simulink model "exp03_sist_integro"  (Simulink 7.7)
settings: Solver=ode23t  StartTime=0.0  StopTime=0.1  RelTol=1e-5
libraries: powerlib x13, powerlib_extras x6
settings Model: Creator=alunos  LastModifiedBy=alunos

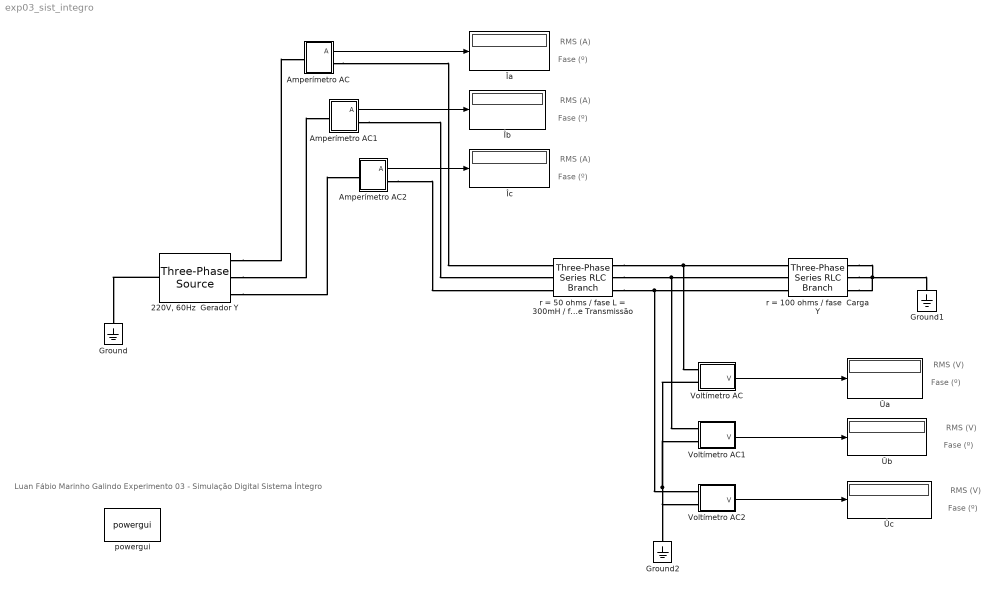
== system exp03_sist_integro ==
  note: RMS (A)
  note: Fase (º)
  note: RMS (A)
  note: Fase (º)
  note: RMS (A)
  note: Fase (º)
  note: RMS (V)
  note: Fase (º)
  note: RMS (V)
  note: Fase (º)
  note: RMS (V)
  note: Fase (º)
  note: Luan Fábio Marinho Galindo
      | Experimento 03 - Simulação Digital
      | Sistema Íntegro
  "220V, 60Hz  Gerador Y" : powerlib/Electrical Sources/Three-Phase Source  SystemSampleTime=-1  Voltage=220  PhaseAngle=90  Frequency=60  InternalConnection=Yn  SpecifyImpedance=off  Resistance=0.001  Inductance=0  ShortCircuitLevel=100e6  BaseVoltage=25e3  XRratio=7  BusType=swing  Pref=0  Qref=0  Qmin=-inf  Qmax=inf
  Amperímetro AC : Subsystem
  Amperímetro AC1 : Subsystem
  Amperímetro AC2 : Subsystem
  Ground : powerlib/Elements/Ground  PhysicalDomain=powersysdomain  SubClassName=unknown  LeftPortType=p1  RightPortType=p1  LConnTagsString=a
  Ground1 : powerlib/Elements/Ground  PhysicalDomain=powersysdomain  SubClassName=unknown  LeftPortType=p1  RightPortType=p1  LConnTagsString=a
  Ground2 : powerlib/Elements/Ground  PhysicalDomain=powersysdomain  SubClassName=unknown  LeftPortType=p1  RightPortType=p1  LConnTagsString=a
  Voltímetro AC : Subsystem
  Voltímetro AC1 : Subsystem
  Voltímetro AC2 : Subsystem
  powergui : powerlib/powergui  Priority=1  SystemSampleTime=-1  SimulationMode=Continuous  SampleTime=50e-6  frequency=60  SPID=off  DisableSnubberDevices=off  DisableRonSwitches=off  DisableVfSwitches=off  SwTol=0  Interpol=off  DisplayEquations=off  FunctionMessages=off  frequencyindice=60  Pbase=100e6  ErrMax=1e-4  Iterations=50  UnitsV=kV  UnitsW=MW  echomessages=off  HookPort=off  EnableUseOfTLC=off  x0status=blocks  RestoreLinks=warning  ResistiveCurrentMeasurement=off  Ylog=off  Xlog=on  ShowGrid=off  save=off  variable=ZData  ZoomFFT=off  StartTime=0.0  cycles=1  DisplayStyle=1  FreqAxis=off  MaxFrequency=1000  frequencyindicesteady=1  display=off  methode=off
  r = 100 ohms / fase  Carga Y : powerlib/Elements/Three-Phase Series RLC Branch  PhysicalDomain=powersysdomain  SubClassName=unknown  LeftPortType=p1  RightPortType=p1  LConnTagsString=A|B|C  RConnTagsString=A|B|C  BranchType=R  Resistance=100  Inductance=1e-3  Capacitance=1e-6  Measurements=None
  r = 50 ohms / fase L = 300mH / fase  Linha de Transmissão : powerlib/Elements/Three-Phase Series RLC Branch  PhysicalDomain=powersysdomain  SubClassName=unknown  LeftPortType=p1  RightPortType=p1  LConnTagsString=A|B|C  RConnTagsString=A|B|C  BranchType=RL  Resistance=50  Inductance=300e-3  Capacitance=1e-6  Measurements=None
  Îa : Display
      settings: Format=bank
  Îb : Display
      settings: Format=bank
  Îc : Display
      settings: Format=bank
  Ûa : Display
      settings: Format=bank
  Ûb : Display
      settings: Format=bank
  Ûc : Display
      settings: Format=bank
  wires:
  Amperímetro AC/1(A) -> Îa/1
  Amperímetro AC1/1(A) -> Îb/1
  Amperímetro AC2/1(A) -> Îc/1
  Voltímetro AC/1(V) -> Ûa/1
  Voltímetro AC1/1(V) -> Ûb/1
  Voltímetro AC2/1(V) -> Ûc/1
  connections:
  "220V, 60Hz  Gerador Y"/RConn1 -- Amperímetro AC/LConn1
  "220V, 60Hz  Gerador Y"/RConn2 -- Amperímetro AC1/LConn1
  "220V, 60Hz  Gerador Y"/RConn3 -- Amperímetro AC2/LConn1
  Amperímetro AC/RConn1 -- r = 50 ohms / fase L = 300mH / fase  Linha de Transmissão/LConn1
  Amperímetro AC1/RConn1 -- r = 50 ohms / fase L = 300mH / fase  Linha de Transmissão/LConn2
  Amperímetro AC2/RConn1 -- r = 50 ohms / fase L = 300mH / fase  Linha de Transmissão/LConn3
  r = 100 ohms / fase  Carga Y/RConn2 -- Ground1/LConn1 -- r = 100 ohms / fase  Carga Y/RConn3 -- r = 100 ohms / fase  Carga Y/RConn1
  r = 50 ohms / fase L = 300mH / fase  Linha de Transmissão/RConn1 -- r = 100 ohms / fase  Carga Y/LConn1 -- Voltímetro AC/LConn1
  r = 50 ohms / fase L = 300mH / fase  Linha de Transmissão/RConn2 -- r = 100 ohms / fase  Carga Y/LConn2 -- Voltímetro AC1/LConn1
  r = 50 ohms / fase L = 300mH / fase  Linha de Transmissão/RConn3 -- r = 100 ohms / fase  Carga Y/LConn3 -- Voltímetro AC2/LConn1
  Voltímetro AC/LConn2 -- Voltímetro AC1/LConn2 -- Ground2/LConn1 -- Voltímetro AC2/LConn2
  "220V, 60Hz  Gerador Y"/LConn1 -- Ground/LConn1

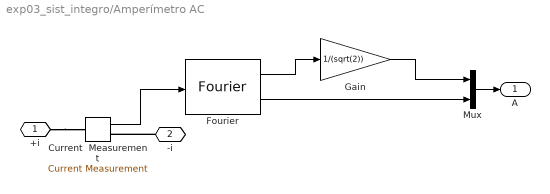
== system exp03_sist_integro/Amperímetro AC ==
  Current  Measurement : powerlib/Measurements/Current Measurement  SystemSampleTime=-1  PhasorSimulation=off  OutputType=Complex  PSBequivalent=0
  Fourier : powerlib_extras/Measurements/Fourier  SystemSampleTime=-1  f1=60  n=1
  Gain : Gain  Gain=1/(sqrt(2))
  Mux : Mux  Inputs=2
  +i : PMIOPort  Port=1  Side=Left
  -i : PMIOPort  Port=2  Side=Right
  A : Outport
  wires:
  Fourier/1 -> Gain/1
  Fourier/2 -> Mux/2
  Gain/1 -> Mux/1
  Current  Measurement/1 -> Fourier/1
  Mux/1 -> A/1
  connections:
  +i/RConn1 -- Current  Measurement/LConn1
  -i/RConn1 -- Current  Measurement/RConn1

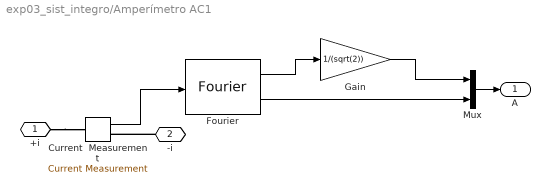
== system exp03_sist_integro/Amperímetro AC1 ==
  Current  Measurement : powerlib/Measurements/Current Measurement  SystemSampleTime=-1  PhasorSimulation=off  OutputType=Complex  PSBequivalent=0
  Fourier : powerlib_extras/Measurements/Fourier  SystemSampleTime=-1  f1=60  n=1
  Gain : Gain  Gain=1/(sqrt(2))
  Mux : Mux  Inputs=2
  +i : PMIOPort  Port=1  Side=Left
  -i : PMIOPort  Port=2  Side=Right
  A : Outport
  wires:
  Fourier/1 -> Gain/1
  Fourier/2 -> Mux/2
  Gain/1 -> Mux/1
  Current  Measurement/1 -> Fourier/1
  Mux/1 -> A/1
  connections:
  +i/RConn1 -- Current  Measurement/LConn1
  -i/RConn1 -- Current  Measurement/RConn1

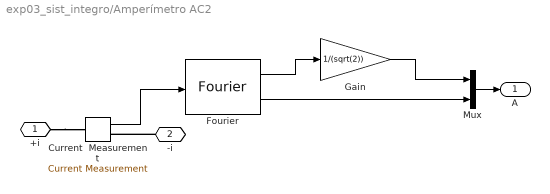
== system exp03_sist_integro/Amperímetro AC2 ==
  Current  Measurement : powerlib/Measurements/Current Measurement  SystemSampleTime=-1  PhasorSimulation=off  OutputType=Complex  PSBequivalent=0
  Fourier : powerlib_extras/Measurements/Fourier  SystemSampleTime=-1  f1=60  n=1
  Gain : Gain  Gain=1/(sqrt(2))
  Mux : Mux  Inputs=2
  +i : PMIOPort  Port=1  Side=Left
  -i : PMIOPort  Port=2  Side=Right
  A : Outport
  wires:
  Fourier/1 -> Gain/1
  Fourier/2 -> Mux/2
  Gain/1 -> Mux/1
  Current  Measurement/1 -> Fourier/1
  Mux/1 -> A/1
  connections:
  +i/RConn1 -- Current  Measurement/LConn1
  -i/RConn1 -- Current  Measurement/RConn1

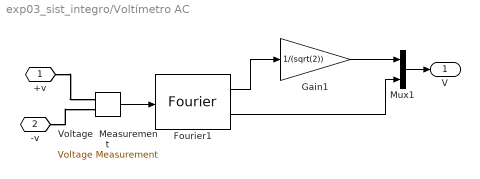
== system exp03_sist_integro/Voltímetro AC ==
  Fourier1 : powerlib_extras/Measurements/Fourier  SystemSampleTime=-1  f1=60  n=1
  Gain1 : Gain  Gain=1/(sqrt(2))
  Mux1 : Mux  Inputs=2
  Voltage  Measurement : powerlib/Measurements/Voltage Measurement  SystemSampleTime=-1  PhasorSimulation=off  OutputType=Complex  PSBequivalent=0
  +v : PMIOPort  Port=1  Side=Left
  -v : PMIOPort  Port=2  Side=Left
  V : Outport
  wires:
  Voltage  Measurement/1 -> Fourier1/1
  Fourier1/1 -> Gain1/1
  Gain1/1 -> Mux1/1
  Fourier1/2 -> Mux1/2
  Mux1/1 -> V/1
  connections:
  +v/RConn1 -- Voltage  Measurement/LConn1
  -v/RConn1 -- Voltage  Measurement/LConn2

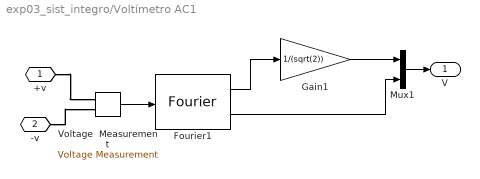
== system exp03_sist_integro/Voltímetro AC1 ==
  Fourier1 : powerlib_extras/Measurements/Fourier  SystemSampleTime=-1  f1=60  n=1
  Gain1 : Gain  Gain=1/(sqrt(2))
  Mux1 : Mux  Inputs=2
  Voltage  Measurement : powerlib/Measurements/Voltage Measurement  SystemSampleTime=-1  PhasorSimulation=off  OutputType=Complex  PSBequivalent=0
  +v : PMIOPort  Port=1  Side=Left
  -v : PMIOPort  Port=2  Side=Left
  V : Outport
  wires:
  Voltage  Measurement/1 -> Fourier1/1
  Fourier1/1 -> Gain1/1
  Gain1/1 -> Mux1/1
  Fourier1/2 -> Mux1/2
  Mux1/1 -> V/1
  connections:
  +v/RConn1 -- Voltage  Measurement/LConn1
  -v/RConn1 -- Voltage  Measurement/LConn2

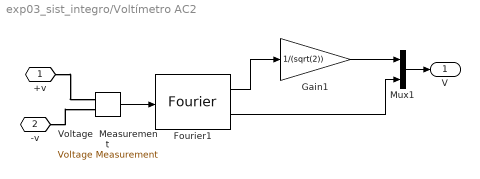
== system exp03_sist_integro/Voltímetro AC2 ==
  Fourier1 : powerlib_extras/Measurements/Fourier  SystemSampleTime=-1  f1=60  n=1
  Gain1 : Gain  Gain=1/(sqrt(2))
  Mux1 : Mux  Inputs=2
  Voltage  Measurement : powerlib/Measurements/Voltage Measurement  SystemSampleTime=-1  PhasorSimulation=off  OutputType=Complex  PSBequivalent=0
  +v : PMIOPort  Port=1  Side=Left
  -v : PMIOPort  Port=2  Side=Left
  V : Outport
  wires:
  Voltage  Measurement/1 -> Fourier1/1
  Fourier1/1 -> Gain1/1
  Gain1/1 -> Mux1/1
  Fourier1/2 -> Mux1/2
  Mux1/1 -> V/1
  connections:
  +v/RConn1 -- Voltage  Measurement/LConn1
  -v/RConn1 -- Voltage  Measurement/LConn2
